simulink model "parte2_eje2_GeneradorSincronoBusInfinito"  (R2017b)
settings: Solver=ode45  StartTime=0.0  StopTime=2  RelTol=1e-3  EnableMultiTasking=on
model workspace (MAT data in the model file):
  D = 0
  F = 60
  H = 6.5
  KAe = 200
  T1e = 1
  T1p = 0.648927607606
  T2e = 10
  T2p = 0.216309202535
  T3 = 1.40659340659
  T3p = 0.648927607606
  T4p = 0.216309202535
  Tee = 0.01
  Tre = 0.01
  Twp = 10
  k1 = 2.21807614913
  k2 = 3.1205207777
  k3 = 0.175824175824
  k4 = 4.68078116655
  k5 = -0.130081858844
  k6 = 0.00523421739465
values from neighbouring files (symbols this model uses):
  K1 = 0.7643    [parte2_ej2_GeneradorBusInfinitoHP.m]    (also in parte2_eje2_HPModel.m = Eb*eqo/D*(RT*sin(do)+XTD*cos(do))+Eb*iqo/D*(xq-xpd)*(XTQ*sin)
  K2 = 0.8649    [parte2_ej2_GeneradorBusInfinitoHP.m]    (also in parte2_eje2_HPModel.m = Lads/(Lads+Lfd)*(RT/D*eqo+(XTQ*(xq-xpd)/D+1)*iqo))
  K3 = 0.3230    (= 0.323)    [parte2_ej2_GeneradorBusInfinitoHP.m]    (also in parte2_eje2_HPModel.m = 0.286464655633)
  K4 = 1.4187    [parte2_ej2_GeneradorBusInfinitoHP.m]    (also in parte2_eje2_HPModel.m = Eb/D*(xd-xpd)*(XTQ*sin(do)-RT*cos(do)))
  K5 = -(vdo/Et)*xq*Eb*cos(do)/(xe+xq)-(vqo/Et)*xpd*Eb*sin(do)/(xe+xpd)    [parte2_eje2_HPModel.m]
  K6 = xe*(vqo/Et)/(xe+xpd)    [parte2_eje2_HPModel.m]
  Kd = 10    [parte2_eje2_HPModel.m]
settings Model: Creator=ramos  LastModifiedBy=cjuar
settings DataIOCC: LimitDataPoints=on  SaveFormat=Array  SignalLoggingSaveFormat=ModelDataLogs
settings OptimizationCC: ExpressionDepthLimit=2147483647  LifeSpan=inf
settings DebuggingCC: UnderspecifiedInitializationDetection=Classic  MergeDetectMultiDrivingBlocksExec=none  SolverPrmCheckMsg=warning  FcnCallInpInsideContextMsg=warning  StateNameClashWarn=warning  SFUnexpectedBacktrackingDiag=warning  SFNoUnconditionalDefaultTransitionDiag=warning  SFExecutionAtInitializationDiag=none
settings HardwareCC: ProdBitPerPointer=32  ProdBitPerSizeT=32  ProdBitPerPtrDiffT=32  ProdLargestAtomicFloat=None  ProdIntDivRoundTo=Undefined  ProdEndianess=Unspecified  ProdWordSize=32  ProdHWDeviceType=32-bit Generic
settings ModelReferenceCC: PropagateSignalLabelsOutOfModel=off
settings CodeAppCC: StateflowObjectComments=on
settings GRTTargetCC: TargetLangStandard=C89/C90 (ANSI)  GeneratePreprocessorConditionals=Disable all  CombineOutputUpdateFcns=off  GRTInterface=on
settings ConfigComp: CovMetricSettings=dw  CovHtmlReporting=on  CovSaveCumulativeToWorkspaceVar=on  CovSaveSingleToWorkspaceVar=on  CovExternalEMLEnable=off

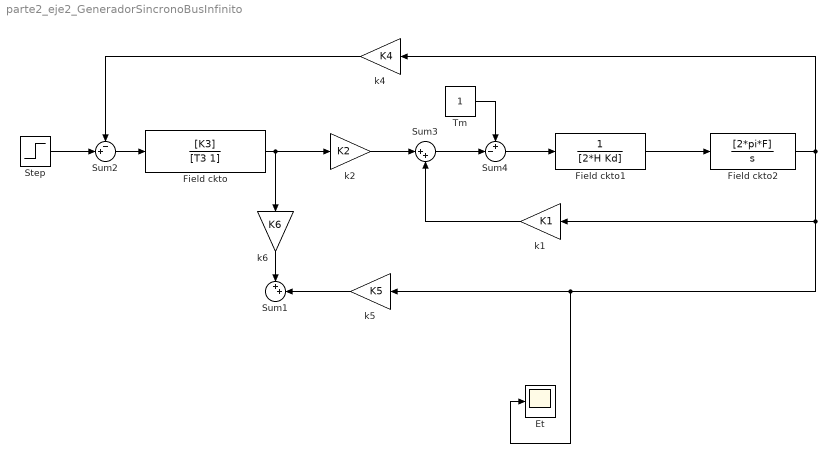
== system parte2_eje2_GeneradorSincronoBusInfinito ==
  Et : Scope
  Field ckto : TransferFcn  Numerator=[K3]  Denominator=[T3 1]
  Field ckto1 : TransferFcn  Denominator=[2*H Kd]
  Field ckto2 : TransferFcn  Numerator=[2*pi*F]  Denominator=[1 0]
  Step : Step  After=0  SampleTime=0
  Sum1 : Sum  Inputs=++|
  Sum2 : Sum  Inputs=-+|
  Sum3 : Sum  Inputs=|++
  Sum4 : Sum  Inputs=+-|
  Tm : Constant
  k1 : Gain  Gain=K1
  k2 : Gain  Gain=K2
  k4 : Gain  Gain=K4
  k5 : Gain  Gain=K5
  k6 : Gain  Gain=K6
  wires:
  Field ckto/1 -> k2/1, k6/1
  k6/1 -> Sum1/1
  Sum2/1 -> Field ckto/1
  k4/1 -> Sum2/1
  k5/1 -> Sum1/2
  k2/1 -> Sum3/1
  k1/1 -> Sum3/2
  Sum3/1 -> Sum4/2
  Tm/1 -> Sum4/1
  Sum4/1 -> Field ckto1/1
  Field ckto1/1 -> Field ckto2/1
  Field ckto2/1 -> k1/1, Et/1, k5/1, k4/1
  Step/1 -> Sum2/2
